simulink model "Pacemaker_Assignment2_group33_Final"  (R2020a)
settings: Solver=FixedStepAuto  StartTime=0.0  StopTime=10.0  FixedStep=1e-3  RelTol=1e-3  EnableMultiTasking=on
undefined symbols (not defined in the file): A0, A1, D0, D1, D10, D11, D12, D13, D2, D3, D4, D5, D6, D7, D8, D9, magnitude, PTA0, PTA1, PTA2, PTB2, PTB23, PTB3, PTB9, PTC16, PTC17, PTC2, PTC3, PTC4, PTD0, PTD1, PTD2, PTD3
libraries: frdmk64flib x21, etargetslib x2, dspstat3 x1
settings Model: ExtModeTrigDuration=5  Creator=sxj  LastModifiedBy=sxj
settings OptimizationCC: EnhancedBackFolding=on  PassReuseOutputArgsAs=Individual arguments  ZeroExternalMemoryAtStartup=off  ZeroInternalMemoryAtStartup=off  MaxStackSize=64  OptimizeBlockOrder=speed  DifferentSizesBufferReuse=on  OptimizationCustomize=off  EfficientTunableParamExpr=on
settings DebuggingCC: ParameterTunabilityLossMsg=error
settings HardwareCC: ProdBitPerPointer=32  ProdBitPerSizeT=32  ProdBitPerPtrDiffT=32  ProdLargestAtomicInteger=Long  ProdLargestAtomicFloat=Double  ProdWordSize=32  ProdHWDeviceType=ARM Compatible->ARM Cortex
settings SFSimCC: MATLABDynamicMemAlloc=off
settings RTWCC: SystemTargetFile=ert.tlc  HardwareBoard=NXP FRDM-K64F  TemplateMakefile=ert_default_tmf  Toolchain=GNU Tools for ARM Embedded Processors
settings CodeAppCC: ForceParamTrailComments=on  IgnoreCustomStorageClasses=off  OperatorAnnotations=on  SimulinkDataObjDesc=on  SFDataObjDesc=on  InsertBlockDesc=on

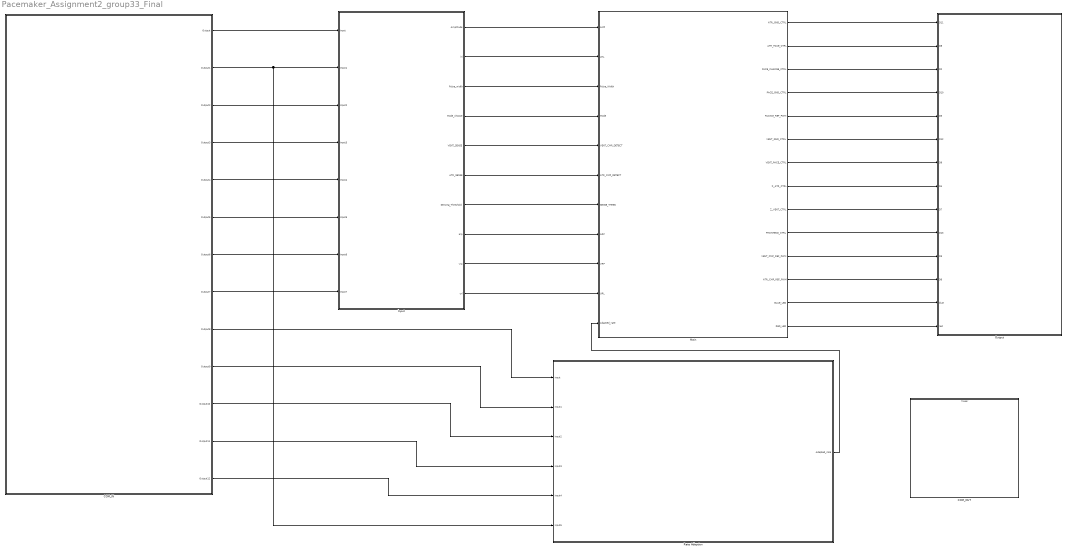
== system Pacemaker_Assignment2_group33_Final ==
  COM_IN : Subsystem
  COM_OUT : Subsystem
  Input : Subsystem
  Main : Stateflow chart  TreatAsAtomicUnit=on
  Output : Subsystem
  Rate Adaption : Subsystem
  wires:
  Input/1(Amplitude) -> Main/1(AMP)
  Input/2(lrl) -> Main/2(LRL)
  Input/3(Pulse_width) -> Main/3(Pulse_Width)
  Input/4(Mode_choose) -> Main/4(Mode)
  Input/5(VENT_SENSE) -> Main/5(VENT_CMP_DETECT)
  Input/6(ATR_SENSE) -> Main/6(ATR_CMP_DETECT)
  Input/7(Sensing_Threshold) -> Main/7(SENSE_THRES)
  Main/1(ATR_GND_CTRL) -> Output/1(D11)
  Main/2(ATR_PACE_CTRL) -> Output/2(D8)
  Main/3(PACE_CHARGE_CTRL) -> Output/3(D2)
  Main/4(PACE_GND_CTRL) -> Output/4(D10)
  Main/5(PACING_REF_PWM) -> Output/5(D5)
  Main/6(VENT_GND_CTRL) -> Output/6(D12)
  Main/7(VENT_PACE_CTRL) -> Output/7(D9)
  Main/8(Z_ATR_CTRL) -> Output/8(D4)
  Main/9(Z_VENT_CTRL) -> Output/9(D7)
  Main/10(FRONTEND_CTRL) -> Output/10(D13)
  Main/11(VENT_CMP_REF_PWM) -> Output/11(D3)
  Main/12(ATR_CMP_REF_PWM) -> Output/12(D6)
  Main/13(BLUE_LED) -> Output/13(blue)
  Main/14(RED_LED) -> Output/14(red)
  Input/8(arp) -> Main/8(ARP)
  Input/9(vrp) -> Main/9(VRP)
  Input/10(url) -> Main/10(URL)
  Rate Adaption/1(Adapted_rate) -> Main/11(Adapted_rate)
  COM_IN/1(Output) -> Input/1(Input)
  COM_IN/2(Output1) -> Rate Adaption/6(Input5), Input/2(Input1)
  COM_IN/3(Output2) -> Input/3(Input2)
  COM_IN/4(Output3) -> Input/4(Input3)
  COM_IN/5(Output4) -> Input/5(Input4)
  COM_IN/6(Output5) -> Input/6(Input5)
  COM_IN/7(Output6) -> Input/7(Input6)
  COM_IN/8(Output7) -> Input/8(Input7)
  COM_IN/9(Output8) -> Rate Adaption/1(Input)
  COM_IN/10(Output9) -> Rate Adaption/2(Input1)
  COM_IN/11(Output10) -> Rate Adaption/3(Input2)
  COM_IN/12(Output11) -> Rate Adaption/4(Input3)
  COM_IN/13(Output12) -> Rate Adaption/5(Input4)

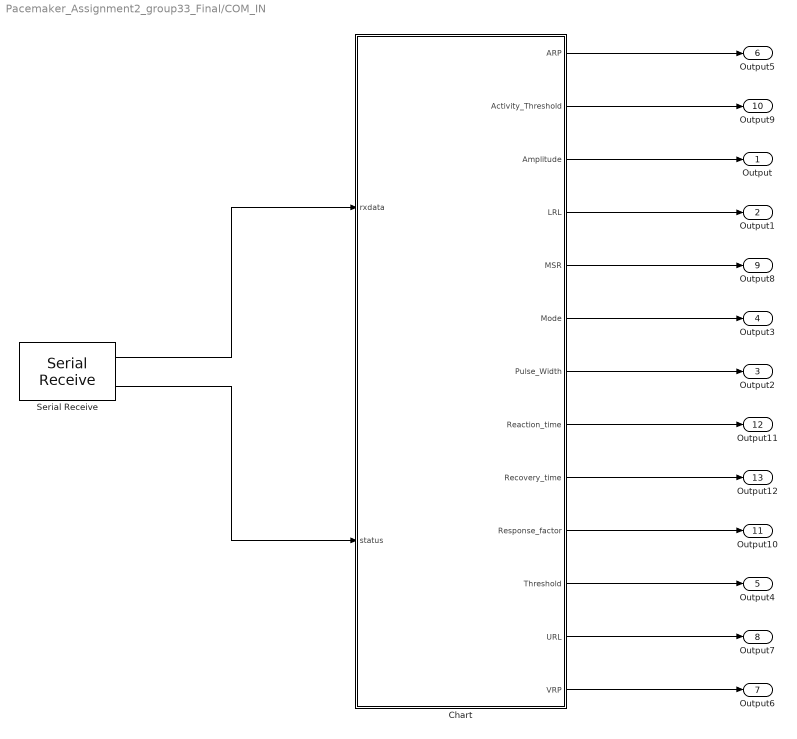
== system Pacemaker_Assignment2_group33_Final/COM_IN ==
  Chart : Stateflow chart  TreatAsAtomicUnit=on
  Serial Receive : frdmk64flib/Serial Receive  SCIModule=0  Baudrate=uint32(9600)  Parity=None  StopBits=1  HardwareFlowControl=None  ByteOrder=LittleEndian  DataType=uint8  DataLength=36  BlockingMode=off  OutputStatus=on  SampleTime=-1
  Output : Outport
  Output1 : Outport  Port=2  OutDataTypeStr=uint16
  Output2 : Outport  Port=3
  Output3 : Outport  Port=4
  Output4 : Outport  Port=5
  Output5 : Outport  Port=6
  Output6 : Outport  Port=7
  Output7 : Outport  Port=8
  Output8 : Outport  Port=9
  Output9 : Outport  Port=10
  Output10 : Outport  Port=11
  Output11 : Outport  Port=12
  Output12 : Outport  Port=13
  wires:
  Serial Receive/1 -> Chart/1(rxdata)
  Chart/1(ARP) -> Output5/1
  Chart/2(Activity_Threshold) -> Output9/1
  Chart/3(Amplitude) -> Output/1
  Chart/4(LRL) -> Output1/1
  Chart/5(MSR) -> Output8/1
  Chart/6(Mode) -> Output3/1
  Chart/7(Pulse_Width) -> Output2/1
  Chart/8(Reaction_time) -> Output11/1
  Chart/9(Recovery_time) -> Output12/1
  Chart/10(Response_factor) -> Output10/1
  Chart/11(Threshold) -> Output4/1
  Chart/12(URL) -> Output7/1
  Chart/13(VRP) -> Output6/1
  Serial Receive/2 -> Chart/2(status)

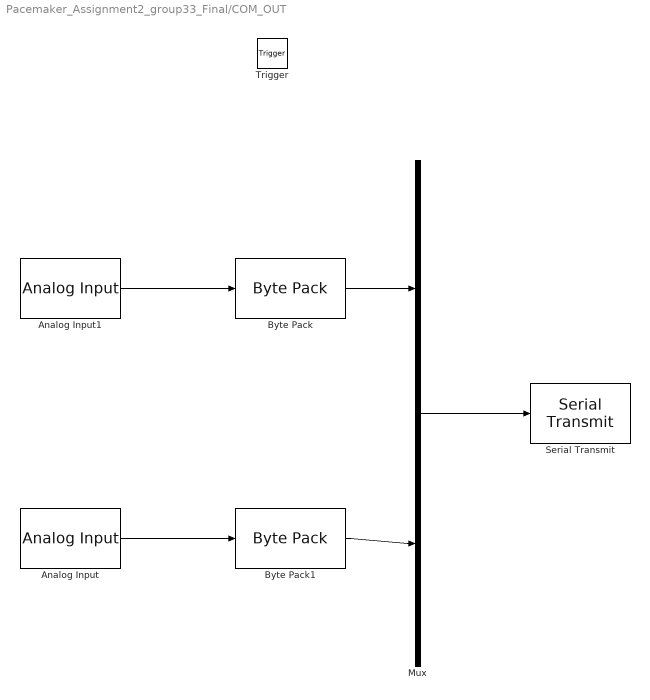
== system Pacemaker_Assignment2_group33_Final/COM_OUT ==
  Trigger : TriggerPort  TriggerType=function-call  IsSimulinkFunction=on  FunctionName=send_params  VariantControl=Variant  PortDimensions=1
  Analog Input : frdmk64flib/Analog Input  Whichpin=PTB3 (A1)  SampleTime=-1
  Analog Input1 : frdmk64flib/Analog Input  Whichpin=PTB2 (A0)  SampleTime=-1
  Byte Pack : etargetslib/Byte Pack  datatypes={'double'}  byteAlign=1
  Byte Pack1 : etargetslib/Byte Pack  datatypes={'double'}  byteAlign=1
  Mux : Mux  Inputs=2
  Serial Transmit : frdmk64flib/Serial Transmit  SCIModule=0  Baudrate=uint32(9600)  Parity=None  StopBits=1  HardwareFlowControl=None  ByteOrder=LittleEndian  BlockingMode=on  OutputStatus=off
  wires:
  Analog Input/1 -> Byte Pack1/1
  Byte Pack/1 -> Mux/1
  Mux/1 -> Serial Transmit/1
  Analog Input1/1 -> Byte Pack/1
  Byte Pack1/1 -> Mux/2

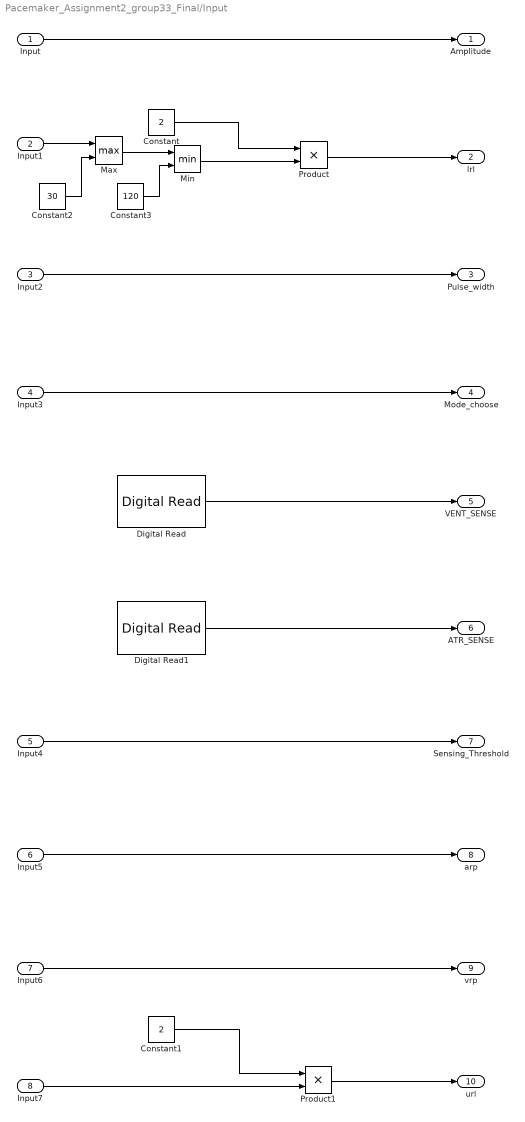
== system Pacemaker_Assignment2_group33_Final/Input ==
  Input : Inport
  Input1 : Inport  Port=2
  Input2 : Inport  Port=3
  Input3 : Inport  Port=4
  Input4 : Inport  Port=5
  Input5 : Inport  Port=6
  Input6 : Inport  Port=7
  Input7 : Inport  Port=8
  Constant : Constant  Value=2
  Constant1 : Constant  Value=2
  Constant2 : Constant  Value=30
  Constant3 : Constant  Value=120
  Digital Read : frdmk64flib/Digital Read  Whichpin=PTC17 (D1)  SampleTime=-1
  Digital Read1 : frdmk64flib/Digital Read  Whichpin=PTC16 (D0)  SampleTime=-1
  Max : MinMax  Function=max  Inputs=2
  Min : MinMax  Inputs=2
  Product : Product
  Product1 : Product  OutDataTypeStr=uint16
  Amplitude : Outport
  lrl : Outport  Port=2
  Pulse_width : Outport  Port=3
  Mode_choose : Outport  Port=4
  VENT_SENSE : Outport  Port=5
  ATR_SENSE : Outport  Port=6
  Sensing_Threshold : Outport  Port=7
  arp : Outport  Port=8
  vrp : Outport  Port=9
  url : Outport  Port=10
  wires:
  Input/1 -> Amplitude/1
  Input3/1 -> Mode_choose/1
  Digital Read/1 -> VENT_SENSE/1
  Digital Read1/1 -> ATR_SENSE/1
  Input4/1 -> Sensing_Threshold/1
  Input5/1 -> arp/1
  Input6/1 -> vrp/1
  Product/1 -> lrl/1
  Product1/1 -> url/1
  Constant/1 -> Product/1
  Input7/1 -> Product1/2
  Constant1/1 -> Product1/1
  Input2/1 -> Pulse_width/1
  Constant2/1 -> Max/2
  Constant3/1 -> Min/2
  Input1/1 -> Max/1
  Max/1 -> Min/1
  Min/1 -> Product/2

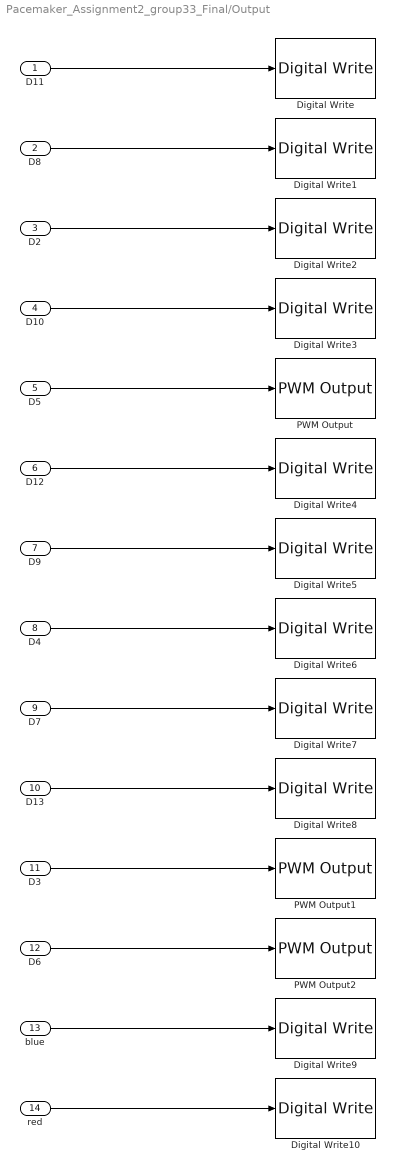
== system Pacemaker_Assignment2_group33_Final/Output ==
  D11 : Inport
  D8 : Inport  Port=2
  D2 : Inport  Port=3
  D10 : Inport  Port=4
  D5 : Inport  Port=5
  D12 : Inport  Port=6
  D9 : Inport  Port=7
  D4 : Inport  Port=8
  D7 : Inport  Port=9
  D13 : Inport  Port=10
  D3 : Inport  Port=11
  D6 : Inport  Port=12
  blue : Inport  Port=13
  red : Inport  Port=14
  Digital Write : frdmk64flib/Digital Write  Whichpin=PTD2 (D11)
  Digital Write1 : frdmk64flib/Digital Write  Whichpin=PTA0 (D8)
  Digital Write10 : frdmk64flib/Digital Write  Whichpin=RED_LED
  Digital Write2 : frdmk64flib/Digital Write  Whichpin=PTB9 (D2)
  Digital Write3 : frdmk64flib/Digital Write  Whichpin=PTD0 (D10)
  Digital Write4 : frdmk64flib/Digital Write  Whichpin=PTD3 (D12)
  Digital Write5 : frdmk64flib/Digital Write  Whichpin=PTC4 (D9)
  Digital Write6 : frdmk64flib/Digital Write  Whichpin=PTB23 (D4)
  Digital Write7 : frdmk64flib/Digital Write  Whichpin=PTC3 (D7)
  Digital Write8 : frdmk64flib/Digital Write  Whichpin=PTD1 (D13)
  Digital Write9 : frdmk64flib/Digital Write  Whichpin=BLUE_LED
  PWM Output : frdmk64flib/PWM Output  Whichpin=PTA2 (D5)  InitialFrequency=2000  InitialDutyCycle=0
  PWM Output1 : frdmk64flib/PWM Output  Whichpin=PTA1 (D3)  InitialFrequency=2000  InitialDutyCycle=0
  PWM Output2 : frdmk64flib/PWM Output  Whichpin=PTC2 (D6)  InitialFrequency=2000  InitialDutyCycle=0
  wires:
  D11/1 -> Digital Write/1
  D8/1 -> Digital Write1/1
  D2/1 -> Digital Write2/1
  D10/1 -> Digital Write3/1
  D5/1 -> PWM Output/1
  D12/1 -> Digital Write4/1
  D9/1 -> Digital Write5/1
  D4/1 -> Digital Write6/1
  D7/1 -> Digital Write7/1
  D13/1 -> Digital Write8/1
  D3/1 -> PWM Output1/1
  D6/1 -> PWM Output2/1
  blue/1 -> Digital Write9/1
  red/1 -> Digital Write10/1

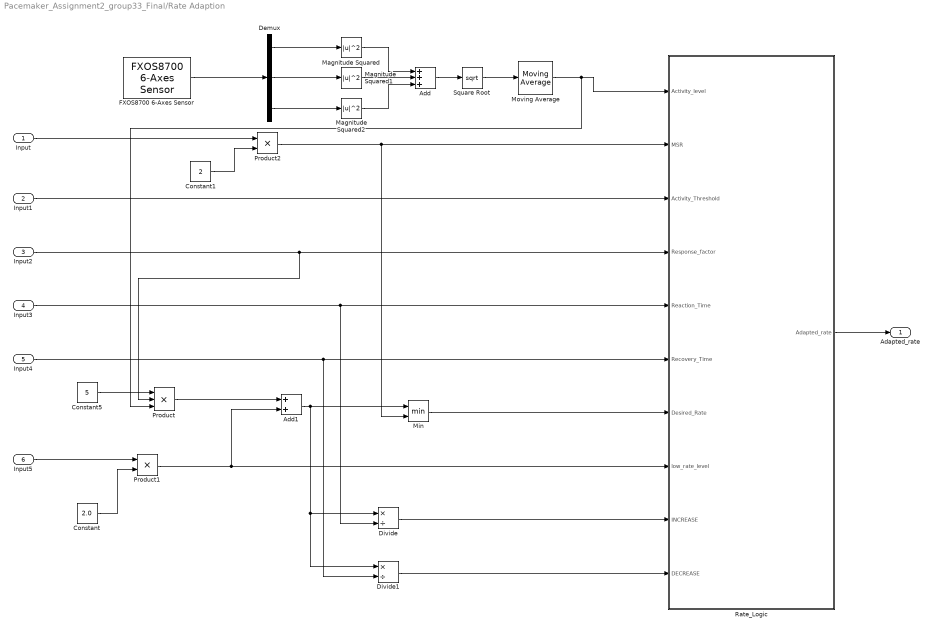
== system Pacemaker_Assignment2_group33_Final/Rate Adaption ==
  Input : Inport
  Input1 : Inport  Port=2
  Input2 : Inport  Port=3
  Input3 : Inport  Port=4
  Input4 : Inport  Port=5
  Input5 : Inport  Port=6  OutDataTypeStr=uint16
  Add : Sum  Inputs=+++
  Add1 : Sum
  Constant : Constant  Value=2.0
  Constant1 : Constant  Value=2
  Constant5 : Constant  Value=5
  Demux : Demux  Outputs=3
  Divide : Product  Inputs=*/
  Divide1 : Product  Inputs=*/
  FXOS8700 6-Axes Sensor : frdmk64flib/FXOS8700 6-Axes Sensor  Activesensor=Accelerometer only  ODR=800Hz  HybridODR=400Hz  Accelfullrange=-4g to +4g  SampleTime=-1
  Magnitude Squared : Math  Operator=magnitude^2  SaturateOnIntegerOverflow=on
  Magnitude Squared1 : Math  Operator=magnitude^2  SaturateOnIntegerOverflow=on
  Magnitude Squared2 : Math  Operator=magnitude^2  SaturateOnIntegerOverflow=on
  Min : MinMax  Inputs=2
  Moving Average : dspstat3/Moving Average  Method=Sliding window  ForgettingFactorPort=off  SpecifyWindowLength=on  WindowLength=100  ForgettingFactor=0.9  SimulateUsing=Code generation
  Product : Product  Inputs=3
  Product1 : Product  OutDataTypeStr=double
  Product2 : Product  OutDataTypeStr=uint8
  Rate_Logic : Stateflow chart  TreatAsAtomicUnit=on
  Square Root : Sqrt  SaturateOnIntegerOverflow=on
  Adapted_rate : Outport
  wires:
  Demux/1 -> Magnitude Squared/1
  Magnitude Squared1/1 -> Add/2
  Add/1 -> Square Root/1
  FXOS8700 6-Axes Sensor/1 -> Demux/1
  Demux/2 -> Magnitude Squared1/1
  Demux/3 -> Magnitude Squared2/1
  Magnitude Squared/1 -> Add/1
  Magnitude Squared2/1 -> Add/3
  Square Root/1 -> Moving Average/1
  Input/1 -> Product2/1
  Input2/1 -> Product/2, Rate_Logic/4(Response_factor)
  Input3/1 -> Divide/2, Rate_Logic/5(Reaction_Time)
  Input4/1 -> Divide1/2, Rate_Logic/6(Recovery_Time)
  Moving Average/1 -> Product/3, Rate_Logic/1(Activity_level)
  Product/1 -> Add1/1
  Product1/1 -> Add1/2, Rate_Logic/8(low_rate_level)
  Add1/1 -> Divide1/1, Divide/1, Min/1
  Min/1 -> Rate_Logic/7(Desired_Rate)
  Divide/1 -> Rate_Logic/9(INCREASE)
  Rate_Logic/1(Adapted_rate) -> Adapted_rate/1
  Constant5/1 -> Product/1
  Divide1/1 -> Rate_Logic/10(DECREASE)
  Input5/1 -> Product1/1
  Product2/1 -> Min/2, Rate_Logic/2(MSR)
  Input1/1 -> Rate_Logic/3(Activity_Threshold)
  Constant/1 -> Product1/2
  Constant1/1 -> Product2/2

== stateflow chart Pacemaker_Assignment2_group33_Final/Rate Adaption/Rate_Logic ==
  state Increase_pend
  state Initialize
    entry:
    Adapted_rate = low_rate_level;
  state Increase_
    entry:
    Adapted_rate = Adapted_rate + INCREASE;
  state Reached_desire
    entry:
    Adapted_rate = Desired_Rate;
  state Inc_Dec
  state Dec_Inc
  state Decrease_
    entry:
    Adapted_rate = Adapted_rate - DECREASE;
  state Decrease_pend
  Increase_pend -> Increase_ : after(Reaction_Time,msec)
  Increase_ -> Increase_pend [order 1] : [Adapted_rate < Desired_Rate]
  (default) -> Initialize
  Initialize -> Initialize [order 2] : [Activity_level <= Activity_Threshold]
  Reached_desire -> Reached_desire [order 2] : [Activity_level > Activity_Threshold]
  Initialize -> Increase_ [order 1] : [Activity_level > Activity_Threshold]
  Increase_ -> Reached_desire [order 2] : [Adapted_rate >= Desired_Rate]
  Increase_ -> Inc_Dec [order 3] : [Activity_level <= Activity_Threshold]
  Dec_Inc -> Increase_ : after(Reaction_Time,msec)
  Decrease_ -> Initialize [order 2] : [Adapted_rate <= low_rate_level]
  Reached_desire -> Decrease_ [order 1] : [Activity_level <= Activity_Threshold]
  Inc_Dec -> Decrease_ : after(Recovery_Time,msec)
  Decrease_ -> Dec_Inc [order 1] : [Activity_level > Activity_Threshold]
  Decrease_ -> Decrease_pend [order 3] : [Adapted_rate > low_rate_level]
  Decrease_pend -> Decrease_ : after(Recovery_Time,msec)
  data: Activity_level input; MSR input uint8; Activity_Threshold input single; Response_factor input uint16; Reaction_Time input uint16; Recovery_Time input uint16; Desired_Rate input; low_rate_level input double; INCREASE input; DECREASE input; Adapted_rate output double

== stateflow chart Pacemaker_Assignment2_group33_Final/COM_IN/Chart ==
  state SEND_PARAM
    entry:
    Mode =typecast(rxdata(3:4),'uint16');
    Amplitude = typecast(rxdata(5:6),'uint16');
    LRL = typecast(rxdata(7:8),'uint16');
    Pulse_Width = typecast(rxdata(9:12),'single');
    Threshold = typecast(rxdata(13:14),'uint16');
    ARP = typecast(rxdata(15:18),'single');
    VRP = typecast(rxdata(19:22),'single');
    URL = typecast(rxdata(23:24),'uint16');
    MSR = typecast(rxdata(25:26),'uint16');
    Activity_Threshold = typecast(rxdata(27:30),'single');
    Response_factor = typecast(rxdata(31:32),'uint16');
    Reaction_time = typecast(rxdata(33:34),'uint16');
    Recovery_time = typecast(rxdata(35:36),'uint16');
  state Initial_State
    entry:
    Mode = 7;
    Amplitude = 100;
    LRL = 60;
    Pulse_Width = 0.4; %4/10 = 0.4
    Threshold = 66;
    ARP = 320; %2 byte
    VRP = 320; %2 byte
    URL = 120; %2 byte
    MSR = 120; %2 byte
    Activity_Threshold = 1.1; %11/10 = 1.1
    Response_factor = 8;
    Reaction_time = 10;
    Recovery_time = 30;
  state STANDBY
  state SEND_BACK
    entry:
    send_params();
  SEND_PARAM -> STANDBY
  (junction 10) -> SEND_PARAM [order 1] : [rxdata(2) == hex2dec('55')]
  (default) -> Initial_State
  (junction 7) -> STANDBY [order 2]
  Initial_State -> STANDBY
  STANDBY -> (junction 7) : [status == 0]
  (junction 7) -> (junction 10) [order 1] : [rxdata(1) == hex2dec('16')]
  (junction 10) -> SEND_BACK [order 2] : [rxdata(2) == hex2dec('22')]
  SEND_BACK -> STANDBY
  data: rxdata input uint8; status input uint8; ARP output single; Activity_Threshold output single; Amplitude output uint16; LRL output uint16; MSR output uint16; Mode output uint16; Pulse_Width output single; Reaction_time output uint16; Recovery_time output uint16; Response_factor output uint16; Threshold output uint16; URL output uint16; VRP output single

== stateflow chart Pacemaker_Assignment2_group33_Final/Main ==
  state AOO
    note: ?
    state AOO_CHARGE
      %State for charging C22 and Discharging C21
      entry:
      PACING_REF_PWM = AMP;
      PACE_CHARGE_CTRL = 1;
      ATR_PACE_CTRL = 0;
      ATR_GND_CTRL = 1;
      PACE_GND_CTRL = 1;
      Z_ATR_CTRL = 0;
      VENT_PACE_CTRL = 0;
      VENT_GND_CTRL = 0;
      Z_VENT_CTRL = 0;
      BLUE_LED = 1;
      RED_LED = 0;
    state AOO_PACE
      %State for pacemaker actual pacing
      entry:
      PACING_REF_PWM = AMP;
      PACE_CHARGE_CTRL = 0;
      ATR_PACE_CTRL = 1;
      ATR_GND_CTRL = 0;
      PACE_GND_CTRL = 1;
      Z_ATR_CTRL = 0;
      VENT_PACE_CTRL = 0;
      VENT_GND_CTRL = 0;
      Z_VENT_CTRL = 0;
      BLUE_LED = 1;
      RED_LED = 0;
    (default) -> AOO_CHARGE
    AOO_CHARGE -> AOO_PACE : [after((60000/LRL)-Pulse_Width,msec)]
    AOO_PACE -> AOO_CHARGE : [after(Pulse_Width,msec)]
  state AOOR
    state AOOR_PACE
      %State for pacemaker actual pacing
      entry:
      PACING_REF_PWM = AMP;
      PACE_CHARGE_CTRL = 0;
      ATR_PACE_CTRL = 1;
      ATR_GND_CTRL = 0;
      PACE_GND_CTRL = 1;
      Z_ATR_CTRL = 0;
      VENT_PACE_CTRL = 0;
      VENT_GND_CTRL = 0;
      Z_VENT_CTRL = 0;
      BLUE_LED = 1;
      RED_LED = 0;
    state AOOR_CHARGE
      %State for charging C22 and Discharging C21
      entry:
      PACING_REF_PWM = AMP;
      PACE_CHARGE_CTRL = 1;
      ATR_PACE_CTRL = 0;
      ATR_GND_CTRL = 1;
      PACE_GND_CTRL = 1;
      Z_ATR_CTRL = 0;
      VENT_PACE_CTRL = 0;
      VENT_GND_CTRL = 0;
      Z_VENT_CTRL = 0;
      BLUE_LED = 0;
      RED_LED = 1;
    (default) -> AOOR_CHARGE
    AOOR_CHARGE -> AOOR_PACE : after(60000/Adapted_rate-Pulse_Width,msec)
    AOOR_PACE -> AOOR_CHARGE : after(Pulse_Width,msec)
  state VVIR
    state VVI_entry
      %Entry State setting variables
      % identical to Charging State
      entry:
      PACING_REF_PWM = AMP;
      PACE_CHARGE_CTRL = 1;
      VENT_PACE_CTRL = 0;
      VENT_GND_CTRL = 1;
      PACE_GND_CTRL = 1;
      Z_VENT_CTRL = 0;
      FRONTEND_CTRL = 1;
      VENT_CMP_REF_PWM = SENSE_THRES;
      ATR_PACE_CTRL = 0;
      ATR_GND_CTRL = 0;
      Z_ATR_CTRL = 0;
    state Sensed
      %Natural activities detected
    state VVI_CHARGE
      %State for charging C22 and Discharging C21
      entry:
      PACING_REF_PWM = AMP;
      PACE_CHARGE_CTRL = 1;
      VENT_PACE_CTRL = 0;
      VENT_GND_CTRL = 1;
      PACE_GND_CTRL = 1;
      Z_VENT_CTRL = 0;
      FRONTEND_CTRL = 1;
      VENT_CMP_REF_PWM = SENSE_THRES;
      ATR_PACE_CTRL = 0;
      ATR_GND_CTRL = 0;
      Z_ATR_CTRL = 0;
    state VVI_Sense
      %Detect Natural activities
    state VVI_PACE
      %State for pacamekr actual pacing
      entry:
      PACING_REF_PWM = AMP;
      PACE_CHARGE_CTRL = 0;
      VENT_PACE_CTRL = 1;
      VENT_GND_CTRL = 0;
      PACE_GND_CTRL = 1;
      Z_VENT_CTRL = 0;
      FRONTEND_CTRL = 1;
      VENT_CMP_REF_PWM = SENSE_THRES;
      ATR_PACE_CTRL = 0;
      ATR_GND_CTRL = 0;
      Z_ATR_CTRL = 0;
    (default) -> VVIR.VVI_entry
    VVIR.Sensed -> VVIR.VVI_Sense : after(VRP,msec)
    VVIR.VVI_entry -> VVIR.VVI_Sense
    VVIR.VVI_Sense -> VVIR.Sensed [order 1] : [VENT_CMP_DETECT == 1]
    VVIR.VVI_Sense -> VVIR.VVI_PACE [order 2] : after((60000/Adapted_rate)-VRP,msec)
    VVIR.VVI_CHARGE -> VVIR.VVI_Sense : after(VRP-Pulse_Width,msec)
    VVIR.VVI_PACE -> VVIR.VVI_CHARGE : after(Pulse_Width,msec)
  state IDLE_STATE
  state VVI
    state VVI_entry
      %Entry State setting variables
      % identical to Charging State
      entry:
      PACING_REF_PWM = AMP;
      PACE_CHARGE_CTRL = 1;
      VENT_PACE_CTRL = 0;
      VENT_GND_CTRL = 1;
      PACE_GND_CTRL = 1;
      Z_VENT_CTRL = 0;
      FRONTEND_CTRL = 1;
      VENT_CMP_REF_PWM = SENSE_THRES;
      ATR_PACE_CTRL = 0;
      ATR_GND_CTRL = 0;
      Z_ATR_CTRL = 0;
    state Sensed
      %Natural activities detected
    state VVI_CHARGE
      %State for charging C22 and Discharging C21
      entry:
      PACING_REF_PWM = AMP;
      PACE_CHARGE_CTRL = 1;
      VENT_PACE_CTRL = 0;
      VENT_GND_CTRL = 1;
      PACE_GND_CTRL = 1;
      Z_VENT_CTRL = 0;
      FRONTEND_CTRL = 1;
      VENT_CMP_REF_PWM = SENSE_THRES;
      ATR_PACE_CTRL = 0;
      ATR_GND_CTRL = 0;
      Z_ATR_CTRL = 0;
    state VVI_Sense
      %Detect Natural activities
    state VVI_PACE
      %State for pacamekr actual pacing
      entry:
      PACING_REF_PWM = AMP;
      PACE_CHARGE_CTRL = 0;
      VENT_PACE_CTRL = 1;
      VENT_GND_CTRL = 0;
      PACE_GND_CTRL = 1;
      Z_VENT_CTRL = 0;
      FRONTEND_CTRL = 1;
      VENT_CMP_REF_PWM = SENSE_THRES;
      ATR_PACE_CTRL = 0;
      ATR_GND_CTRL = 0;
      Z_ATR_CTRL = 0;
    (default) -> VVI.VVI_entry
    VVI.Sensed -> VVI.VVI_Sense : after(VRP,msec)
    VVI.VVI_entry -> VVI.VVI_Sense
    VVI.VVI_Sense -> VVI.Sensed [order 1] : [VENT_CMP_DETECT == 1]
    VVI.VVI_Sense -> VVI.VVI_PACE [order 2] : after((60000/LRL)-VRP,msec)
    VVI.VVI_CHARGE -> VVI.VVI_Sense : after(VRP-Pulse_Width,msec)
    VVI.VVI_PACE -> VVI.VVI_CHARGE : after(Pulse_Width,msec)
  state AAI
    state AAI_entry
      %Entry State setting variables
      % identical to Charging State
      entry:
      PACING_REF_PWM = AMP;
      PACE_CHARGE_CTRL = 1;
      ATR_PACE_CTRL = 0;
      ATR_GND_CTRL = 1;
      PACE_GND_CTRL = 1;
      Z_ATR_CTRL = 0;
      FRONTEND_CTRL = 1;
      ATR_CMP_REF_PWM = SENSE_THRES;
      VENT_PACE_CTRL = 0;
      VENT_GND_CTRL = 0;
      Z_VENT_CTRL = 0;
    state AAI_Sensed
      %Nastural actvites Detected
    state AAI_PACE
      %State for pacamekr actual pacing
      entry:
      PACING_REF_PWM = AMP;
      PACE_CHARGE_CTRL = 0;
      ATR_PACE_CTRL = 1;
      ATR_GND_CTRL = 0;
      PACE_GND_CTRL = 1;
      Z_ATR_CTRL = 0;
      FRONTEND_CTRL = 1;
      ATR_CMP_REF_PWM = SENSE_THRES;
      VENT_PACE_CTRL = 0;
      VENT_GND_CTRL = 0;
      Z_VENT_CTRL = 0;
    state AAI_CHARGE
      %State for charging C22 and Discharging C21
      entry:
      PACING_REF_PWM = AMP;
      PACE_CHARGE_CTRL = 1;
      ATR_PACE_CTRL = 0;
      ATR_GND_CTRL = 1;
      PACE_GND_CTRL = 1;
      Z_ATR_CTRL = 0;
      FRONTEND_CTRL = 1;
      ATR_CMP_REF_PWM = SENSE_THRES;
      VENT_PACE_CTRL = 0;
      VENT_GND_CTRL = 0;
      Z_VENT_CTRL = 0;
    state AAI_Sense
      %Detect Natural activities
    AAI.AAI_entry -> AAI.AAI_Sense
    AAI.AAI_Sensed -> AAI.AAI_Sense : after(ARP,msec)
    (default) -> AAI.AAI_CHARGE
    AAI.AAI_Sense -> AAI.AAI_Sensed [order 1] : [ATR_CMP_DETECT == 1]
    AAI.AAI_CHARGE -> AAI.AAI_Sense : after(ARP-Pulse_Width,msec)
    AAI.AAI_Sense -> AAI.AAI_PACE [order 2] : after((60000/LRL)-ARP,msec)
    AAI.AAI_PACE -> AAI.AAI_CHARGE : after(Pulse_Width,msec)
  state AAIR
    state AAI_entry
      %Entry State setting variables
      % identical to Charging State
      entry:
      PACING_REF_PWM = AMP;
      PACE_CHARGE_CTRL = 1;
      ATR_PACE_CTRL = 0;
      ATR_GND_CTRL = 1;
      PACE_GND_CTRL = 1;
      Z_ATR_CTRL = 0;
      FRONTEND_CTRL = 1;
      ATR_CMP_REF_PWM = SENSE_THRES;
      VENT_PACE_CTRL = 0;
      VENT_GND_CTRL = 0;
      Z_VENT_CTRL = 0;
    state AAI_Sensed
      %Nastural actvites Detected
    state AAI_PACE
      %State for pacamekr actual pacing
      entry:
      PACING_REF_PWM = AMP;
      PACE_CHARGE_CTRL = 0;
      ATR_PACE_CTRL = 1;
      ATR_GND_CTRL = 0;
      PACE_GND_CTRL = 1;
      Z_ATR_CTRL = 0;
      FRONTEND_CTRL = 1;
      ATR_CMP_REF_PWM = SENSE_THRES;
      VENT_PACE_CTRL = 0;
      VENT_GND_CTRL = 0;
      Z_VENT_CTRL = 0;
    state AAI_CHARGE
      %State for charging C22 and Discharging C21
      entry:
      PACING_REF_PWM = AMP;
      PACE_CHARGE_CTRL = 1;
      ATR_PACE_CTRL = 0;
      ATR_GND_CTRL = 1;
      PACE_GND_CTRL = 1;
      Z_ATR_CTRL = 0;
      FRONTEND_CTRL = 1;
      ATR_CMP_REF_PWM = SENSE_THRES;
      VENT_PACE_CTRL = 0;
      VENT_GND_CTRL = 0;
      Z_VENT_CTRL = 0;
    state AAI_Sense
      %Detect Natural activities
    (default) -> AAIR.AAI_entry
    AAIR.AAI_entry -> AAIR.AAI_Sense
    AAIR.AAI_Sensed -> AAIR.AAI_Sense : after(ARP,msec)
    AAIR.AAI_Sense -> AAIR.AAI_Sensed [order 1] : [ATR_CMP_DETECT == 1]
    AAIR.AAI_CHARGE -> AAIR.AAI_Sense : after(ARP-Pulse_Width,msec)
    AAIR.AAI_Sense -> AAIR.AAI_PACE [order 2] : after((60000/Adapted_rate)-ARP,msec)
    AAIR.AAI_PACE -> AAIR.AAI_CHARGE : after(Pulse_Width,msec)
  state VOOR
    state VOO_PACE
      %State for pacemaker actual pacing
      entry:
      PACING_REF_PWM = AMP;
      PACE_CHARGE_CTRL = 0;
      VENT_PACE_CTRL = 1;
      VENT_GND_CTRL = 0;
      PACE_GND_CTRL = 1;
      Z_VENT_CTRL = 0;
      ATR_PACE_CTRL = 0;
      ATR_GND_CTRL = 0;
      Z_ATR_CTRL = 0;
      BLUE_LED = 1;
      RED_LED = 0;
    state VOO_CHARGE
      %State for charging C22 and Discharging C21
      entry:
      PACING_REF_PWM = AMP;
      PACE_CHARGE_CTRL = 1;
      VENT_PACE_CTRL = 0;
      VENT_GND_CTRL = 1;
      PACE_GND_CTRL = 1;
      Z_VENT_CTRL = 0;
      ATR_PACE_CTRL = 0;
      ATR_GND_CTRL = 0;
      Z_ATR_CTRL = 0;
      BLUE_LED = 0;
      RED_LED = 1;
    (default) -> VOOR.VOO_CHARGE
    VOOR.VOO_CHARGE -> VOOR.VOO_PACE : after(60000/Adapted_rate-Pulse_Width,msec)
    VOOR.VOO_PACE -> VOOR.VOO_CHARGE : after(Pulse_Width,msec)
  state VOO
    state VOO_CHARGE
      %State for charging C22 and Discharging C21
      entry:
      PACING_REF_PWM = AMP;
      PACE_CHARGE_CTRL = 1;
      VENT_PACE_CTRL = 0;
      VENT_GND_CTRL = 1;
      PACE_GND_CTRL = 1;
      Z_VENT_CTRL = 0;
      ATR_PACE_CTRL = 0;
      ATR_GND_CTRL = 0;
      Z_ATR_CTRL = 0;
      BLUE_LED = 0;
      RED_LED = 1;
    state VOO_PACE
      %State for pacemaker actual pacing
      entry:
      PACING_REF_PWM = AMP;
      PACE_CHARGE_CTRL = 0;
      VENT_PACE_CTRL = 1;
      VENT_GND_CTRL = 0;
      PACE_GND_CTRL = 1;
      Z_VENT_CTRL = 0;
      ATR_PACE_CTRL = 0;
      ATR_GND_CTRL = 0;
      Z_ATR_CTRL = 0;
      BLUE_LED = 0;
      RED_LED = 1;
    (default) -> VOO.VOO_CHARGE
    VOO.VOO_CHARGE -> VOO.VOO_PACE : after((60000/LRL)-Pulse_Width,msec)
    VOO.VOO_PACE -> VOO.VOO_CHARGE : after(Pulse_Width,msec)
  IDLE_STATE -> AOO [order 1] : [Mode == 0]
  AOO -> IDLE_STATE : [Mode ~= 0]
  IDLE_STATE -> AOOR [order 5] : [Mode == 4]
  AOOR -> IDLE_STATE : [Mode ~= 4]
  IDLE_STATE -> VVIR [order 8] : [Mode == 7]
  VVIR -> IDLE_STATE : [Mode ~= 7]
  (default) -> IDLE_STATE
  IDLE_STATE -> VVI [order 4] : [Mode == 3]
  IDLE_STATE -> AAI [order 3] : [Mode == 2]
  AAI -> IDLE_STATE : [Mode ~= 2]
  VVI -> IDLE_STATE : [Mode ~= 3]
  IDLE_STATE -> AAIR [order 7] : [Mode == 6]
  AAIR -> IDLE_STATE : [Mode ~= 6]
  IDLE_STATE -> VOOR [order 6] : [Mode == 5]
  IDLE_STATE -> VOO [order 2] : [Mode == 1]
  VOO -> IDLE_STATE : [Mode ~= 1]
  VOOR -> IDLE_STATE : [Mode ~= 5]
  data: AMP input uint16; ATR_GND_CTRL output; ATR_PACE_CTRL output; PACE_CHARGE_CTRL output; PACE_GND_CTRL output; PACING_REF_PWM output; VENT_GND_CTRL output; VENT_PACE_CTRL output; Z_ATR_CTRL output; Z_VENT_CTRL output; LRL input; Pulse_Width input single; Mode input uint16; FRONTEND_CTRL output; VENT_CMP_DETECT input; ATR_CMP_DETECT input; SENSE_THRES input uint16; VENT_CMP_REF_PWM output; ATR_CMP_REF_PWM output; BLUE_LED output; RED_LED output; ARP input single; VRP input single; URL input uint16; Adapted_rate input
